simulink model "Citation_2017a"  (R2017a)
settings: Solver=ode5  StartTime=0.0  StopTime=inf  FixedStep=0.01  RelTol=1e-3  EnableMultiTasking=on
InitFcn:
  | initcit
values from neighbouring files (symbols this model uses):
  aeroinit = [dp_ini;inicoef('CX0');inicoef('CXa');inicoef('CXa2');inicoef('CXq')     ;inicoef('CXde');inicoef('CY0');inicoef('CYB');inicoef('CYp');inicoef('CYr')     ;inicoef('CYda');inicoef('CYdr');inicoef('CZ0');inicoef('CZa');inicoef('CZq')     ;inicoef('CZde');inicoef('Cl0');inicoef('ClB');inicoef('Clp');inicoef('Clr')     ;inicoef('Clda');inicoef('Cldr');inicoef('Cm0');inicoef('Cma');inicoef('Cmq')     ; ...(+113 chars)    [initcit.m]
  Clda_thresh = 3.410e-2/2    (= 0.01705)    [initcit.m]
  h_l_old = zeros(6,sample_size)    [initcit.m]
  h_m_old = zeros(4,sample_size)    [initcit.m]
  h_n_old = zeros(6,sample_size)    [initcit.m]
  h_X_old = zeros(5,sample_size)    [initcit.m]
  h_Y_old = zeros(6,sample_size)    [initcit.m]
  h_Z_old = zeros(4,sample_size)    [initcit.m]
  I = [massinit(5),0, -massinit(8);0, massinit(6),0;-massinit(8),0, massinit(7)]    [initcit.m]
  p_l = [inicoef('Cl0');inicoef('ClB');inicoef('Clp');inicoef('Clr')     ;inicoef('Clda');inicoef('Cldr')].*ones(6,sample_size)    [initcit.m]
  p_m = [inicoef('Cm0');inicoef('Cma');inicoef('Cmq')     ;inicoef('Cmde')].*ones(4,sample_size)    [initcit.m]
  p_n = [inicoef('Cn0');inicoef('CnB');inicoef('Cnp');inicoef('Cnr')     ;inicoef('Cnda');inicoef('Cndr')].*ones(6,sample_size)    [initcit.m]
  p_X = [inicoef('CX0');inicoef('CXa');inicoef('CXa2');inicoef('CXq')     ;inicoef('CXde')].*ones(5,sample_size)    [initcit.m]
  p_Y = [inicoef('CY0');inicoef('CYB');inicoef('CYp');inicoef('CYr')     ;inicoef('CYda');inicoef('CYdr')].*ones(6,sample_size)    [initcit.m]
  p_Z = [inicoef('CZ0');inicoef('CZa');inicoef('CZq')     ;inicoef('CZde')].*ones(4,sample_size)    [initcit.m]
  Pcov_l = 10000*eye(6)    [initcit.m]
  Pcov_m = 10000*eye(4)    [initcit.m]
  Pcov_n = 10000*eye(6)    [initcit.m]
  Pcov_X = 10000*eye(5)    [initcit.m]
  Pcov_Y = 10000*eye(6)    [initcit.m]
  Pcov_Z = 10000*eye(4)    [initcit.m]
  replay = 0    [initcit.m]
  T0 = 288.15    [rho_test.m]
  timeend = inputsim.data{1}.Values.Time(end)    [initcit.m]
  Vw915 = 0    [initcit.m]
  winddir = 45*(pi/180)    (= 0.785398163397)    [initcit.m]
  x0 = []    [cessnac550_3d_sfnc.m]    (also in sfunxyauto.m)
  y_l = zeros(1,sample_size)    [initcit.m]
  y_l_est_old = zeros(size(y_l))    [initcit.m]
  y_m = zeros(1,sample_size)    [initcit.m]
  y_m_est_old = zeros(size(y_m))    [initcit.m]
  y_n = zeros(1,sample_size)    [initcit.m]
  y_n_est_old = zeros(size(y_n))    [initcit.m]
  y_X = zeros(1,sample_size)    [initcit.m]
  y_X_est_old = zeros(size(y_X))    [initcit.m]
  y_Y = zeros(1,sample_size)    [initcit.m]
  y_Y_est_old = zeros(size(y_Y))    [initcit.m]
  y_Z = zeros(1,sample_size)    [initcit.m]
  y_Z_est_old = zeros(size(y_Z))    [initcit.m]
undefined symbols (not defined in the file or in its folder): chord, cv1, cv2, cv3, cv4, deltagmax1, deltagmax2, deltagmax3, deltagmax4, Deng, ealphag, ealphas, g0, hDME, hGS, kt1, kt2, kt3, lh, massinit, matbuaf, matdaf, matdam, matdbbf, matdeaf, matdgaf, matdqaf, matduaf, matdwaw, matedhr, mateif, matelhr, matemhr, matemv1, matemv2, matemve, matetam, mateuaf, matfaaf, matfaxl, matff, matibaf, matibmh, matipaf, matipmh, matiraf, matiuaf, matiwaf, matlaf, matlam, matleaf, matleam, matlgaf, matlqaf, matluaf, matmaaf, matmaam, matmaf, matmam, matmbbf ... (+74)
undefined symbols (not defined in the file): matibb
libraries: simulink x13, templibrary x6, vrlib x1
(part 3 of 7)

== system Citation_2017a/Cessna Citation 500/Citation model DASMAT/AIRCRAFT MODEL ==
  ua : Inport
  ut : Inport  Port=2
  massinit : Inport  Port=3
  Environment : Inport  Port=4
  AFM : Subsystem
  AIRDATA : Subsystem
  Demux : Demux  Outputs=[8 1]
  EFM : Subsystem
  EQM : Subsystem
  FM SORT : Subsystem
  GRAVITY : Subsystem
  LANDING GEAR : Subsystem
  OBSERVATIONS : Subsystem
  WIND/TURBULENCE : Subsystem
  x : Outport
  xdot : Outport  Port=2
  yatm : Outport  Port=3
  yad1 : Outport  Port=4
  yad2 : Outport  Port=5
  wind : Outport  Port=6
  gust : Outport  Port=7
  yacc : Outport  Port=8
  yfp : Outport  Port=9
  ys : Outport  Port=10
  FMa : Outport  Port=11
  FMag : Outport  Port=12
  FMt : Outport  Port=13
  ypp : Outport  Port=14
  wires:
  AFM/1(FMa) -> FM SORT/1(FMa), EQM/2(FMa)
  OBSERVATIONS/3(ys) -> ys/1
  OBSERVATIONS/2(yfp) -> yfp/1
  EQM/4(FMtot corrected) -> OBSERVATIONS/4(FMtot)
  EQM/3(yuvw) -> OBSERVATIONS/3(yuvw)
  EFM/1(FMt) -> FM SORT/3(FMt), FMt/1
  AFM/4(FMag) -> FM SORT/2(FMag), FMag/1
  ua/1 -> AFM/2(ua), LANDING GEAR/4(ua)
  ut/1 -> EFM/2(ut)
  OBSERVATIONS/1(yacc) -> yacc/1
  FM SORT/1(FMtot) -> EQM/1("FMtot ")
  EQM/5(FMa corrected) -> OBSERVATIONS/5(FMa), FMa/1
  AFM/2(FMadot) -> EQM/3(FMadot)
  AFM/3(FMbdot) -> EQM/4(FMbdot)
  GRAVITY/1(Fgr) -> FM SORT/4("Fgr "), OBSERVATIONS/6(Fgr)
  massinit/1 -> EFM/3(massinit), AFM/3(massinit), GRAVITY/2(massinit), EQM/5(massinit), OBSERVATIONS/7(massinit), LANDING GEAR/3(massinit)
  AIRDATA/3(yad2) -> EFM/6(yad2), AFM/5(yad2), yad2/1
  AIRDATA/2(yad1) -> AFM/4(yad1), EFM/5(yad1), yad1/1
  AIRDATA/1(yatm) -> yatm/1, GRAVITY/3(yatm), OBSERVATIONS/8(yatm), EFM/4(yatm), AFM/7(yatm)
  EQM/1(x) -> GRAVITY/1("x "), LANDING GEAR/1(x), EFM/1(x), AFM/1(x), WIND/TURBULENCE/1("x "), AIRDATA/1(x), x/1, OBSERVATIONS/1(x)
  WIND/TURBULENCE/1(wind) -> EQM/6(wind), wind/1
  EQM/2(xdot) -> xdot/1, OBSERVATIONS/2(xdot), LANDING GEAR/2(xdot)
  Environment/1 -> Demux/1
  Demux/1 -> gust/1, AFM/6(gust)
  Demux/2 -> AIRDATA/2(terrain elevation), LANDING GEAR/5(terr elev)  "terrain elevation"
  LANDING GEAR/1(Fmt) -> FM SORT/5(Fgear)
  EFM/2(ypp) -> ypp/1

== system Citation_2017a/Controllers/ANDI rotational rate controller/Linear Controller ==
  e_omega : Inport
  int reset : Inport  Port=2
  Demux : Demux  Outputs=3
  Mux : Mux  Inputs=3
  PID Controller : simulink/Continuous/PID Controller  Controller=PID  TimeDomain=Continuous-time  SampleTime=-1  IntegratorMethod=Forward Euler  FilterMethod=Forward Euler  Form=Parallel  UseFilter=on  ControllerParametersSource=internal  P=10  I=1  D=0  N=100  InitialConditionSource=internal  InitialConditionForIntegrator=0  InitialConditionForFilter=0  ExternalReset=rising  LimitOutput=off  UpperSaturationLimit=inf  LowerSaturationLimit=-inf  LinearizeAsGain=on  AntiWindupMode=none  Kb=1  TrackingMode=off  Kt=1  PParamMin=[]  PParamMax=[]  IParamMin=[]  IParamMax=[]  DParamMin=[]  DParamMax=[]  NParamMin=[]  NParamMax=[]  KbParamMin=[]  KbParamMax=[]  KtParamMin=[]  KtParamMax=[]  POutMin=[]  POutMax=[]  IOutMin=[]  IOutMax=[]  DOutMin=[]  DOutMax=[]  NOutMin=[]  NOutMax=[]  KbOutMin=[]  KbOutMax=[]  KtOutMin=[]  KtOutMax=[]  IntegratorOutMin=[]  IntegratorOutMax=[]  FilterOutMin=[]  FilterOutMax=[]  SumOutMin=[]  SumOutMax=[]  SumI1OutMin=[]  SumI1OutMax=[]  SumI2OutMin=[]  SumI2OutMax=[]  SumI3OutMin=[]  SumI3OutMax=[]  SumDOutMin=[]  SumDOutMax=[]  SaturationOutMin=[]  SaturationOutMax=[]  IntegratorContinuousStateAttributes=''  IntegratorStateMustResolveToSignalObject=off  IntegratorRTWStateStorageClass=Auto  FilterContinuousStateAttributes=''  FilterStateMustResolveToSignalObject=off  FilterRTWStateStorageClass=Auto  DifferentiatorICPrevScaledInput=0  DifferentiatorOutMin=[]  DifferentiatorOutMax=[]
  PID Controller1 : simulink/Continuous/PID Controller  Controller=PID  TimeDomain=Continuous-time  SampleTime=-1  IntegratorMethod=Forward Euler  FilterMethod=Forward Euler  Form=Parallel  UseFilter=on  ControllerParametersSource=internal  P=10  I=2  D=0  N=1  InitialConditionSource=internal  InitialConditionForIntegrator=0  InitialConditionForFilter=0  ExternalReset=rising  LimitOutput=off  UpperSaturationLimit=inf  LowerSaturationLimit=-inf  LinearizeAsGain=on  AntiWindupMode=none  Kb=1  TrackingMode=off  Kt=1  PParamMin=[]  PParamMax=[]  IParamMin=[]  IParamMax=[]  DParamMin=[]  DParamMax=[]  NParamMin=[]  NParamMax=[]  KbParamMin=[]  KbParamMax=[]  KtParamMin=[]  KtParamMax=[]  POutMin=[]  POutMax=[]  IOutMin=[]  IOutMax=[]  DOutMin=[]  DOutMax=[]  NOutMin=[]  NOutMax=[]  KbOutMin=[]  KbOutMax=[]  KtOutMin=[]  KtOutMax=[]  IntegratorOutMin=[]  IntegratorOutMax=[]  FilterOutMin=[]  FilterOutMax=[]  SumOutMin=[]  SumOutMax=[]  SumI1OutMin=[]  SumI1OutMax=[]  SumI2OutMin=[]  SumI2OutMax=[]  SumI3OutMin=[]  SumI3OutMax=[]  SumDOutMin=[]  SumDOutMax=[]  SaturationOutMin=[]  SaturationOutMax=[]  IntegratorContinuousStateAttributes=''  IntegratorStateMustResolveToSignalObject=off  IntegratorRTWStateStorageClass=Auto  FilterContinuousStateAttributes=''  FilterStateMustResolveToSignalObject=off  FilterRTWStateStorageClass=Auto  DifferentiatorICPrevScaledInput=0  DifferentiatorOutMin=[]  DifferentiatorOutMax=[]
  PID Controller2 : simulink/Continuous/PID Controller  Controller=PID  TimeDomain=Continuous-time  SampleTime=-1  IntegratorMethod=Forward Euler  FilterMethod=Forward Euler  Form=Parallel  UseFilter=on  ControllerParametersSource=internal  P=8  I=2  D=0  N=1  InitialConditionSource=internal  InitialConditionForIntegrator=0  InitialConditionForFilter=0  ExternalReset=rising  LimitOutput=off  UpperSaturationLimit=inf  LowerSaturationLimit=-inf  LinearizeAsGain=on  AntiWindupMode=none  Kb=1  TrackingMode=off  Kt=1  PParamMin=[]  PParamMax=[]  IParamMin=[]  IParamMax=[]  DParamMin=[]  DParamMax=[]  NParamMin=[]  NParamMax=[]  KbParamMin=[]  KbParamMax=[]  KtParamMin=[]  KtParamMax=[]  POutMin=[]  POutMax=[]  IOutMin=[]  IOutMax=[]  DOutMin=[]  DOutMax=[]  NOutMin=[]  NOutMax=[]  KbOutMin=[]  KbOutMax=[]  KtOutMin=[]  KtOutMax=[]  IntegratorOutMin=[]  IntegratorOutMax=[]  FilterOutMin=[]  FilterOutMax=[]  SumOutMin=[]  SumOutMax=[]  SumI1OutMin=[]  SumI1OutMax=[]  SumI2OutMin=[]  SumI2OutMax=[]  SumI3OutMin=[]  SumI3OutMax=[]  SumDOutMin=[]  SumDOutMax=[]  SaturationOutMin=[]  SaturationOutMax=[]  IntegratorContinuousStateAttributes=''  IntegratorStateMustResolveToSignalObject=off  IntegratorRTWStateStorageClass=Auto  FilterContinuousStateAttributes=''  FilterStateMustResolveToSignalObject=off  FilterRTWStateStorageClass=Auto  DifferentiatorICPrevScaledInput=0  DifferentiatorOutMin=[]  DifferentiatorOutMax=[]
  v : Outport
  wires:
  Demux/1 -> PID Controller1/1
  PID Controller2/1 -> Mux/3  "vr"
  PID Controller/1 -> Mux/2  "vq"
  Demux/3 -> PID Controller2/1
  PID Controller1/1 -> Mux/1  "vp"
  Demux/2 -> PID Controller/1
  Mux/1 -> v/1
  e_omega/1 -> Demux/1
  int reset/1 -> PID Controller/2, PID Controller2/2, PID Controller1/2

== system Citation_2017a/Controllers/Default Actuator Control/Yaw damper1 ==
  state : Inport
  inputs : Inport  Port=2
  Gain : Gain  SaturateOnIntegerOverflow=on  OutDataTypeStr=Inherit: Same as input  ParamDataTypeStr=Inherit: Same as input
  Washout : TransferFcn  Numerator=[1 0]  Denominator=[1 1/4]
  dr : Gain  Gain=[0 0 1 0 0 0 0 0 0 0]  SaturateOnIntegerOverflow=on  OutDataTypeStr=Inherit: Same as input  ParamDataTypeStr=Inherit: Same as input
  not used : Terminator
  r  sel : Selector  IndexOptions=Index vector (dialog)  Indices=[3]  OutputSizes=1
  controller output : Outport
  wires:
  Washout/1 -> Gain/1
  dr/1 -> controller output/1
  state/1 -> r  sel/1
  r  sel/1 -> Washout/1  "r"
  inputs/1 -> not used/1
  Gain/1 -> dr/1

== system Citation_2017a/Controllers/Default Actuator Control/auto throttle1 ==
  state : Inport
  inputs : Inport  Port=2
  Gain : Gain  Gain=0.5  SaturateOnIntegerOverflow=on  OutDataTypeStr=Inherit: Same as input  ParamDataTypeStr=Inherit: Same as input
  Saturation : Saturate  UpperLimit=1.0  LowerLimit=0.0
  Sum : Sum  Inputs=+-|  SaturateOnIntegerOverflow=on
  VTAS ref (trim value) : Constant  Value=x0(4)
  VTAS sel : Selector  IndexOptions=Index vector (dialog)  Indices=[4]  OutputSizes=1
  controller output is later added to pilot input! : Sum  Inputs=|+-  SaturateOnIntegerOverflow=on
  pla1&2 : Gain  Gain=[0 0 0 0 0 0 0 0 1 1]  SaturateOnIntegerOverflow=on  OutDataTypeStr=Inherit: Same as input  ParamDataTypeStr=Inherit: Same as input
  pla1&2 as well : Gain  Gain=[0 0 0 0 0 0 0 0 1 1]  SaturateOnIntegerOverflow=on  OutDataTypeStr=Inherit: Same as input  ParamDataTypeStr=Inherit: Same as input
  controller output : Outport
  wires:
  inputs/1 -> pla1&2 as well/1
  state/1 -> VTAS sel/1
  VTAS sel/1 -> Sum/2  "VTAS"
  VTAS ref (trim value)/1 -> Sum/1
  Sum/1 -> Gain/1
  pla1&2/1 -> controller output is later added to pilot input!/1
  Gain/1 -> Saturation/1
  controller output is later added to pilot input!/1 -> controller output/1
  Saturation/1 -> pla1&2/1
  pla1&2 as well/1 -> controller output is later added to pilot input!/2

== system Citation_2017a/Controllers/INDI rotational rate controller/Linear Controller ==
  e_omega : Inport
  int reset : Inport  Port=2
  Demux : Demux  Outputs=3
  Mux : Mux  Inputs=3
  PID Controller : simulink/Continuous/PID Controller  Controller=PID  TimeDomain=Continuous-time  SampleTime=-1  IntegratorMethod=Forward Euler  FilterMethod=Forward Euler  Form=Parallel  UseFilter=on  ControllerParametersSource=internal  P=10  I=1  D=0  N=100  InitialConditionSource=internal  InitialConditionForIntegrator=0  InitialConditionForFilter=0  ExternalReset=rising  LimitOutput=off  UpperSaturationLimit=inf  LowerSaturationLimit=-inf  LinearizeAsGain=on  AntiWindupMode=none  Kb=1  TrackingMode=off  Kt=1  PParamMin=[]  PParamMax=[]  IParamMin=[]  IParamMax=[]  DParamMin=[]  DParamMax=[]  NParamMin=[]  NParamMax=[]  KbParamMin=[]  KbParamMax=[]  KtParamMin=[]  KtParamMax=[]  POutMin=[]  POutMax=[]  IOutMin=[]  IOutMax=[]  DOutMin=[]  DOutMax=[]  NOutMin=[]  NOutMax=[]  KbOutMin=[]  KbOutMax=[]  KtOutMin=[]  KtOutMax=[]  IntegratorOutMin=[]  IntegratorOutMax=[]  FilterOutMin=[]  FilterOutMax=[]  SumOutMin=[]  SumOutMax=[]  SumI1OutMin=[]  SumI1OutMax=[]  SumI2OutMin=[]  SumI2OutMax=[]  SumI3OutMin=[]  SumI3OutMax=[]  SumDOutMin=[]  SumDOutMax=[]  SaturationOutMin=[]  SaturationOutMax=[]  IntegratorContinuousStateAttributes=''  IntegratorStateMustResolveToSignalObject=off  IntegratorRTWStateStorageClass=Auto  FilterContinuousStateAttributes=''  FilterStateMustResolveToSignalObject=off  FilterRTWStateStorageClass=Auto  DifferentiatorICPrevScaledInput=0  DifferentiatorOutMin=[]  DifferentiatorOutMax=[]
  PID Controller1 : simulink/Continuous/PID Controller  Controller=PID  TimeDomain=Continuous-time  SampleTime=-1  IntegratorMethod=Forward Euler  FilterMethod=Forward Euler  Form=Parallel  UseFilter=on  ControllerParametersSource=internal  P=10  I=2  D=0  N=1  InitialConditionSource=internal  InitialConditionForIntegrator=0  InitialConditionForFilter=0  ExternalReset=rising  LimitOutput=off  UpperSaturationLimit=inf  LowerSaturationLimit=-inf  LinearizeAsGain=on  AntiWindupMode=none  Kb=1  TrackingMode=off  Kt=1  PParamMin=[]  PParamMax=[]  IParamMin=[]  IParamMax=[]  DParamMin=[]  DParamMax=[]  NParamMin=[]  NParamMax=[]  KbParamMin=[]  KbParamMax=[]  KtParamMin=[]  KtParamMax=[]  POutMin=[]  POutMax=[]  IOutMin=[]  IOutMax=[]  DOutMin=[]  DOutMax=[]  NOutMin=[]  NOutMax=[]  KbOutMin=[]  KbOutMax=[]  KtOutMin=[]  KtOutMax=[]  IntegratorOutMin=[]  IntegratorOutMax=[]  FilterOutMin=[]  FilterOutMax=[]  SumOutMin=[]  SumOutMax=[]  SumI1OutMin=[]  SumI1OutMax=[]  SumI2OutMin=[]  SumI2OutMax=[]  SumI3OutMin=[]  SumI3OutMax=[]  SumDOutMin=[]  SumDOutMax=[]  SaturationOutMin=[]  SaturationOutMax=[]  IntegratorContinuousStateAttributes=''  IntegratorStateMustResolveToSignalObject=off  IntegratorRTWStateStorageClass=Auto  FilterContinuousStateAttributes=''  FilterStateMustResolveToSignalObject=off  FilterRTWStateStorageClass=Auto  DifferentiatorICPrevScaledInput=0  DifferentiatorOutMin=[]  DifferentiatorOutMax=[]
  PID Controller2 : simulink/Continuous/PID Controller  Controller=PID  TimeDomain=Continuous-time  SampleTime=-1  IntegratorMethod=Forward Euler  FilterMethod=Forward Euler  Form=Parallel  UseFilter=on  ControllerParametersSource=internal  P=8  I=2  D=0  N=1  InitialConditionSource=internal  InitialConditionForIntegrator=0  InitialConditionForFilter=0  ExternalReset=rising  LimitOutput=off  UpperSaturationLimit=inf  LowerSaturationLimit=-inf  LinearizeAsGain=on  AntiWindupMode=none  Kb=1  TrackingMode=off  Kt=1  PParamMin=[]  PParamMax=[]  IParamMin=[]  IParamMax=[]  DParamMin=[]  DParamMax=[]  NParamMin=[]  NParamMax=[]  KbParamMin=[]  KbParamMax=[]  KtParamMin=[]  KtParamMax=[]  POutMin=[]  POutMax=[]  IOutMin=[]  IOutMax=[]  DOutMin=[]  DOutMax=[]  NOutMin=[]  NOutMax=[]  KbOutMin=[]  KbOutMax=[]  KtOutMin=[]  KtOutMax=[]  IntegratorOutMin=[]  IntegratorOutMax=[]  FilterOutMin=[]  FilterOutMax=[]  SumOutMin=[]  SumOutMax=[]  SumI1OutMin=[]  SumI1OutMax=[]  SumI2OutMin=[]  SumI2OutMax=[]  SumI3OutMin=[]  SumI3OutMax=[]  SumDOutMin=[]  SumDOutMax=[]  SaturationOutMin=[]  SaturationOutMax=[]  IntegratorContinuousStateAttributes=''  IntegratorStateMustResolveToSignalObject=off  IntegratorRTWStateStorageClass=Auto  FilterContinuousStateAttributes=''  FilterStateMustResolveToSignalObject=off  FilterRTWStateStorageClass=Auto  DifferentiatorICPrevScaledInput=0  DifferentiatorOutMin=[]  DifferentiatorOutMax=[]
  v : Outport
  wires:
  Demux/1 -> PID Controller1/1
  PID Controller2/1 -> Mux/3  "vr"
  PID Controller/1 -> Mux/2  "vq"
  Demux/3 -> PID Controller2/1
  PID Controller1/1 -> Mux/1  "vp"
  Demux/2 -> PID Controller/1
  Mux/1 -> v/1
  e_omega/1 -> Demux/1
  int reset/1 -> PID Controller/2, PID Controller2/2, PID Controller1/2

== system Citation_2017a/Flight Monitoring/3D Display/Position ==
  Mux2 : Mux  Inputs=3
  x : Constant  Value=0
  y : Constant  Value=0
  z : Constant  Value=0
  Out1 : Outport
  wires:
  y/1 -> Mux2/2
  z/1 -> Mux2/3
  x/1 -> Mux2/1
  Mux2/1 -> Out1/1

== system Citation_2017a/Pilot/Joystick/DualShock ==
  note: Apply Dead zone
  note: Currently configured for a Sony Dualshock 3 Playstation 3 Controller
  JoyStick input : Inport
  "Add deadzone " : Subsystem
  Add deadzone 1 : Subsystem
  Add deadzone 2 : Subsystem
  Add deadzone 3 : Subsystem
  Constant{,1..3} (4 alike) : Constant  Value=0
  Constant{4..7} (4 alike) : Constant  Value=0.05
  Dead Zone{,1..3} (4 alike) : DeadZone  LowerValue=-0.05  UpperValue=0.05  SaturateOnIntegerOverflow=on
  Demux : Demux  Outputs=[5 10]
  Demux1 : Demux  Outputs=5
  Demux2 : Demux  Outputs=[2 1 7]
  Display{,1..3} (4 alike) : Display
  Gain{,1..3} (4 alike) : Gain  Gain=-1  SaturateOnIntegerOverflow=on  OutDataTypeStr=Inherit: Same as input  ParamDataTypeStr=Inherit: Same as input
  Gain11 : Gain  Gain=pi/180  SaturateOnIntegerOverflow=on  OutDataTypeStr=Inherit: Same as input  ParamDataTypeStr=Inherit: Same as input
  Gain4 : Gain  Gain=37.24  SaturateOnIntegerOverflow=on  OutDataTypeStr=Inherit: Same as input  ParamDataTypeStr=Inherit: Same as input
  Gain5 : Gain  Gain=20  SaturateOnIntegerOverflow=on  OutDataTypeStr=Inherit: Same as input  ParamDataTypeStr=Inherit: Same as input
  Gain6 : Gain  SaturateOnIntegerOverflow=on  OutDataTypeStr=Inherit: Same as input  ParamDataTypeStr=Inherit: Same as input
  Gain7 : Gain  Gain=22  SaturateOnIntegerOverflow=on  OutDataTypeStr=Inherit: Same as input  ParamDataTypeStr=Inherit: Same as input
  Gain8 : Gain  Gain=pi/180  SaturateOnIntegerOverflow=on  OutDataTypeStr=Inherit: Same as input  ParamDataTypeStr=Inherit: Same as input
  Gain9 : Gain  Gain=pi/180  SaturateOnIntegerOverflow=on  OutDataTypeStr=Inherit: Same as input  ParamDataTypeStr=Inherit: Same as input
  Mux : Mux  Inputs=5
  Sum{,1..3} (4 alike) : Sum  Inputs=-+|  SaturateOnIntegerOverflow=on
  Terminator : Terminator
  Terminator1 : Terminator
  Terminator2 : Terminator
  "Model Input " : Outport
  wires:
  Gain3/1 -> Gain7/1
  Constant4/1 -> "Add deadzone "/1("Value ")
  Gain4/1 -> Gain8/1
  Constant5/1 -> Add deadzone 3/1("Value ")
  Constant/1 -> Sum/1
  Sum3/1 -> Dead Zone2/1
  "Add deadzone "/1(Out1) -> Gain/1
  Demux1/3 -> Terminator/1
  Demux1/4 -> Sum3/2
  Dead Zone/1 -> "Add deadzone "/2("Input ")
  Sum2/1 -> Dead Zone3/1
  Gain8/1 -> Mux/1, Display/1
  Dead Zone1/1 -> Add deadzone 1/2("Input ")
  Demux1/5 -> Sum1/2
  Add deadzone 1/1(Out1) -> Gain1/1
  Add deadzone 3/1(Out1) -> Gain3/1
  Constant1/1 -> Sum1/1
  Demux1/2 -> Sum2/2
  Gain5/1 -> Gain9/1
  Gain11/1 -> Mux/4, Display3/1
  Constant3/1 -> Sum3/1
  Gain1/1 -> Gain5/1
  Dead Zone2/1 -> Add deadzone 3/2("Input ")
  Add deadzone 2/1(Out1) -> Gain2/1
  Gain/1 -> Gain4/1
  Dead Zone3/1 -> Add deadzone 2/2("Input ")
  Sum/1 -> Dead Zone/1
  Gain9/1 -> Mux/2, Display2/1
  Constant7/1 -> Add deadzone 1/1("Value ")
  Constant6/1 -> Add deadzone 2/1("Value ")
  Sum1/1 -> Dead Zone1/1
  Gain6/1 -> Mux/3, Display1/1
  Gain7/1 -> Gain11/1
  Demux1/1 -> Sum/2
  Constant2/1 -> Sum2/1
  Gain2/1 -> Gain6/1
  JoyStick input/1 -> Demux/1
  Demux2/3 -> Terminator2/1
  Demux/2 -> Demux2/1  "buttons"
  Demux2/1 -> Terminator1/1
  Demux/1 -> Demux1/1
  Mux/1 -> "Model Input "/1
  Demux2/2 -> Mux/5

== system Citation_2017a/Pilot/Joystick/Logitech 3D Pro ==
  note: Apply real actuator limits
  note: Normalize inputs
  note: Apply Dead zone
  note: apply real limits
      | [deg]
      | [%]
  note: normalize inputs
      | aileron [-1,0,1] left+
      | elevator [-1,0,1] forward+
      | rudder [-1,0,1] left+
      | throttle [-1,0,1] forward+
  note: Convert to radians
      | [rad]
      | [%]
  note: raw inputs
      | aileron [-0.6328,0.014,0.72] right+
      | elevator [-0.6973,-0.033,0.5725] backwards+
      | throttle [-0.6407,0,0.5317]bacwards+
      | rudder [-0.56,0.127,0.73] right+
  note: Currently configured for a Logitech Xtreme 3D Pro Joystick
  "JoyStick Input " : Inport
  Constant{,1..3} (4 alike) : Constant  Value=0
  Dead Zone : DeadZone  LowerValue=-0.2  UpperValue=0.2  SaturateOnIntegerOverflow=on
  Dead Zone1 : DeadZone  LowerValue=-0.008  UpperValue=0.008  SaturateOnIntegerOverflow=on
  Dead Zone2 : DeadZone  LowerValue=-0.05  UpperValue=0.05  SaturateOnIntegerOverflow=on
  Dead Zone3 : DeadZone  LowerValue=0  UpperValue=0  SaturateOnIntegerOverflow=on
  Demux : Demux  Outputs=[1 1 2 1 1 2 1 1 1 1]
  Demux1 : Demux
  Demux2 : Demux  Outputs=[4 12]
  Gain : Gain  Gain=-1/0.8  SaturateOnIntegerOverflow=on  OutDataTypeStr=Inherit: Same as input  ParamDataTypeStr=Inherit: Same as input
  Gain1 : Gain  Gain=-1/0.992  SaturateOnIntegerOverflow=on  OutDataTypeStr=Inherit: Same as input  ParamDataTypeStr=Inherit: Same as input
  Gain11 : Gain  Gain=pi/180  SaturateOnIntegerOverflow=on  OutDataTypeStr=Inherit: Same as input  ParamDataTypeStr=Inherit: Same as input
  Gain2 : Gain  Gain=-1  SaturateOnIntegerOverflow=on  OutDataTypeStr=Inherit: Same as input  ParamDataTypeStr=Inherit: Same as input
  Gain3 : Gain  Gain=-1/0.95  SaturateOnIntegerOverflow=on  OutDataTypeStr=Inherit: Same as input  ParamDataTypeStr=Inherit: Same as input
  Gain4 : Gain  Gain=37.24  SaturateOnIntegerOverflow=on  OutDataTypeStr=Inherit: Same as input  ParamDataTypeStr=Inherit: Same as input
  Gain5 : Gain  Gain=20  SaturateOnIntegerOverflow=on  OutDataTypeStr=Inherit: Same as input  ParamDataTypeStr=Inherit: Same as input
  Gain6 : Gain  SaturateOnIntegerOverflow=on  OutDataTypeStr=Inherit: Same as input  ParamDataTypeStr=Inherit: Same as input
  Gain7 : Gain  Gain=22  SaturateOnIntegerOverflow=on  OutDataTypeStr=Inherit: Same as input  ParamDataTypeStr=Inherit: Same as input
  Gain8 : Gain  Gain=pi/180  SaturateOnIntegerOverflow=on  OutDataTypeStr=Inherit: Same as input  ParamDataTypeStr=Inherit: Same as input
  Gain9 : Gain  Gain=pi/180  SaturateOnIntegerOverflow=on  OutDataTypeStr=Inherit: Same as input  ParamDataTypeStr=Inherit: Same as input
  Mux : Mux  Inputs=11
  Sum{,1..3} (4 alike) : Sum  Inputs=-+|  SaturateOnIntegerOverflow=on
  Terminator1 : Terminator
  Terminator2 : Terminator
  Terminator3 : Terminator
  Model Input : Outport
  wires:
  Constant1/1 -> Sum1/1
  Sum2/1 -> Dead Zone3/1
  Sum/1 -> Dead Zone/1
  Dead Zone/1 -> Gain/1
  Dead Zone2/1 -> Gain3/1
  Dead Zone3/1 -> Gain2/1
  Gain5/1 -> Gain9/1
  Gain7/1 -> Gain11/1
  Dead Zone1/1 -> Gain1/1
  Constant2/1 -> Sum2/1
  Sum1/1 -> Dead Zone1/1
  Sum3/1 -> Dead Zone2/1
  Gain4/1 -> Gain8/1
  Demux1/1 -> Sum/2
  Gain1/1 -> Gain5/1
  Constant/1 -> Sum/1
  Demux2/1 -> Demux1/1  "axes"
  Gain3/1 -> Gain7/1
  Constant3/1 -> Sum3/1
  Gain2/1 -> Gain6/1
  Gain/1 -> Gain4/1
  Demux1/3 -> Sum3/2
  Demux1/2 -> Sum1/2
  Demux1/4 -> Sum2/2
  Gain9/1 -> Mux/2  "elevator"
  Gain6/1 -> Mux/3  "thrust"
  Demux/6 -> Terminator2/1
  Demux/1 -> Terminator1/1
  Demux/4 -> Mux/5  "failure button"
  Demux2/2 -> Demux/1  "buttons"
  "JoyStick Input "/1 -> Demux2/1
  Mux/1 -> Model Input/1
  Gain8/1 -> Mux/1  "aileron"
  Gain11/1 -> Mux/4  "rudder"
  Demux/9 -> Mux/8  "Default mode"
  Demux/7 -> Mux/6  "classical rate toggle"
  Demux/10 -> Mux/9  "NDI toggle"
  Demux/8 -> Mux/7  "INDI toggle"
  Demux/3 -> Terminator3/1
  Demux/2 -> Mux/10  "Manual integral reset"
  Demux/5 -> Mux/11  "AT toggle"

== system Citation_2017a/Pilot/Joystick/Stop sim when replay has ended ==
  In1 : Inport
  Clock : Clock
      settings: Decimation=2
  Constant2 : Constant  Value=inf
  Constant3 : Constant  Value=timeend
  Display : Display
  Fcn : Fcn  Expr=u<0
  Stop Simulation : Stop
  Sum1 : Sum  Inputs=|+-
  Switch : Switch  Criteria=u2 > Threshold
  wires:
  Switch/1 -> Sum1/1
  Constant3/1 -> Switch/1
  Fcn/1 -> Stop Simulation/1
  Sum1/1 -> Display/1, Fcn/1
  In1/1 -> Switch/2
  Constant2/1 -> Switch/3
  Clock/1 -> Sum1/2

== system Citation_2017a/Pilot/Joystick/load pre-recorded inputs ==
  From Workspace : FromWorkspace  Commented=on  VariableName=inputsim.data{1}.Values  SampleTime=0
  From Workspace1 : FromWorkspace  Commented=on  VariableName=inputsim.data{3}.Values  SampleTime=0
  From Workspace10 : FromWorkspace  Commented=on  VariableName=inputsim.data{12}.Values  SampleTime=0
  From Workspace11 : FromWorkspace  Commented=on  VariableName=inputsim.data{10}.Values  SampleTime=0
  From Workspace12 : FromWorkspace  Commented=on  VariableName=inputsim.data{11}.Values  SampleTime=0
  From Workspace13 : FromWorkspace  Commented=on  VariableName=inputsim.data{14}.Values  SampleTime=0
  From Workspace14 : FromWorkspace  Commented=on  VariableName=inputsim.data{13}.Values  SampleTime=0
  From Workspace15 : FromWorkspace  Commented=on  VariableName=inputsim.data{16}.Values  SampleTime=0
  From Workspace16 : FromWorkspace  VariableName=joydata  SampleTime=0
  From Workspace2 : FromWorkspace  Commented=on  VariableName=inputsim.data{4}.Values  SampleTime=0
  From Workspace3 : FromWorkspace  Commented=on  VariableName=inputsim.data{5}.Values  SampleTime=0
  From Workspace4 : FromWorkspace  Commented=on  VariableName=inputsim.data{6}.Values  SampleTime=0
  From Workspace5 : FromWorkspace  Commented=on  VariableName=inputsim.data{7}.Values  SampleTime=0
  From Workspace6 : FromWorkspace  Commented=on  VariableName=inputsim.data{8}.Values  SampleTime=0
  From Workspace7 : FromWorkspace  Commented=on  VariableName=inputsim.data{9}.Values  SampleTime=0
  From Workspace8 : FromWorkspace  Commented=on  VariableName=inputsim.data{2}.Values  SampleTime=0
  From Workspace9 : FromWorkspace  Commented=on  VariableName=inputsim.data{15}.Values  SampleTime=0
  Mux : Mux  Commented=on  Inputs=16
  Out1 : Outport
  wires:
  From Workspace/1 -> Mux/1
  From Workspace8/1 -> Mux/2
  From Workspace1/1 -> Mux/3
  From Workspace2/1 -> Mux/4
  From Workspace3/1 -> Mux/5
  From Workspace4/1 -> Mux/6
  From Workspace5/1 -> Mux/7
  From Workspace6/1 -> Mux/8
  From Workspace7/1 -> Mux/9
  From Workspace11/1 -> Mux/10
  From Workspace12/1 -> Mux/11
  From Workspace10/1 -> Mux/12
  From Workspace14/1 -> Mux/13
  From Workspace13/1 -> Mux/14
  From Workspace9/1 -> Mux/15
  From Workspace15/1 -> Mux/16
  From Workspace16/1 -> Out1/1

== system Citation_2017a/Pilot/Select new mode/Triggered Subsystem ==
  note: default mode is the initial condition
  triggers : Inport
  Trigger : TriggerPort  TriggerType=either  VariantControl=Variant
  MATLAB Function : MATLAB Function  TreatAsAtomicUnit=on
  Memory : Memory  X0=zeros(4,1)  InheritSampleTime=on
  Memory1 : Memory  X0=4  InheritSampleTime=on
  index : Outport
  wires:
  triggers/1 -> MATLAB Function/2(triggers)
  MATLAB Function/1(index) -> Memory1/1, index/1
  MATLAB Function/2(triggers_pref) -> Memory/1
  Memory/1 -> MATLAB Function/3("triggers_pref ")
  Memory1/1 -> MATLAB Function/1("index ")

== system Citation_2017a/Cessna Citation 500/Citation model DASMAT/AIRCRAFT MODEL/AFM ==
  x : Inport
  ua : Inport  Port=2
  massinit : Inport  Port=3
  yad1 : Inport  Port=4
  yad2 : Inport  Port=5
  gust : Inport  Port=6
  yatm : Inport  Port=7
  Aero axes-cg transformation : Subsystem
  Aeromod : Subsystem
  FMaerodims : Subsystem
  FMgustdims : Subsystem
  Gust axes-cg transformation : Subsystem
  FMa : Outport
  FMadot : Outport  Port=2
  FMbdot : Outport  Port=3
  FMag : Outport  Port=4
  wires:
  FMaerodims/3(FMbdot) -> FMbdot/1
  FMgustdims/1(FMag) -> FMag/1
  FMaerodims/2(FMadot) -> FMadot/1
  FMaerodims/1(FMa) -> FMa/1
  ua/1 -> Aeromod/2(ua)
  yad2/1 -> Aeromod/5(yad2)
  gust/1 -> Aeromod/6(gust)
  Aero axes-cg transformation/1(Ca) -> FMaerodims/1(Ca)
  Aero axes-cg transformation/2(Cadot) -> FMaerodims/2(Cadot)
  Aero axes-cg transformation/3(Cbdot) -> FMaerodims/3(Cbdot)
  Gust axes-cg transformation/1(Cag) -> FMgustdims/1(Cag)
  yad1/1 -> FMaerodims/5(yad1), FMgustdims/2(yad1), Aeromod/4(yad1)
  massinit/1 -> Aero axes-cg transformation/5(massinit), Gust axes-cg transformation/3(massinit), Aeromod/3(massinit)
  Aeromod/1(Ca) -> Aero axes-cg transformation/1(Ca model)
  Aeromod/2(Cadot) -> Aero axes-cg transformation/2(Cadot model)
  Aeromod/3(Cbdot) -> Aero axes-cg transformation/3(Cbdot model)
  Aeromod/4(Cag) -> Gust axes-cg transformation/1(Cag model)
  x/1 -> Aero axes-cg transformation/4("x "), Gust axes-cg transformation/2("x "), FMaerodims/4(x), Aeromod/1(x)
  yatm/1 -> Aeromod/7(yatm)

== system Citation_2017a/Cessna Citation 500/Citation model DASMAT/AIRCRAFT MODEL/AIRDATA ==
  x : Inport
  terrain elevation : Inport  Port=2
  Demux : Demux  Outputs=[8 2 8]
  Demux1 : Demux  Outputs=[5 1 2]
  Mux : Mux  Inputs=[5 1 2]
  Sum : Sum  Inputs=-+|  SaturateOnIntegerOverflow=on
  airdata : S-Function  FunctionName=ac_atmos  SFunctionDeploymentMode=off  EnableBusSupport=off
  yatm : Outport
  yad1 : Outport  Port=2
  yad2 : Outport  Port=3
  wires:
  x/1 -> airdata/1
  airdata/1 -> Demux/1
  Demux/2 -> yad1/1
  Demux/3 -> yad2/1
  Demux/1 -> Demux1/1
  Mux/1 -> yatm/1
  Demux1/1 -> Mux/1
  Demux1/3 -> Mux/3
  Demux1/2 -> Sum/2
  Sum/1 -> Mux/2
  terrain elevation/1 -> Sum/1

== system Citation_2017a/Cessna Citation 500/Citation model DASMAT/AIRCRAFT MODEL/EFM ==
  x : Inport
  ut : Inport  Port=2
  massinit : Inport  Port=3
  yatm : Inport  Port=4
  yad1 : Inport  Port=5
  yad2 : Inport  Port=6
  Engine axes-cg transformation : Subsystem
  Engmod : Subsystem
  FMt : Outport
  ypp : Outport  Port=2
  wires:
  massinit/1 -> Engine axes-cg transformation/3(massinit)
  Engine axes-cg transformation/1(FMt) -> FMt/1
  ut/1 -> Engmod/2(ut)
  yatm/1 -> Engmod/3(yatm)
  yad2/1 -> Engmod/5(yad2)
  x/1 -> Engine axes-cg transformation/2("x "), Engmod/1(x)
  yad1/1 -> Engmod/4(yad1)
  Engmod/1(FMt) -> Engine axes-cg transformation/1(FMt model)
  Engmod/2(ypp) -> ypp/1

== system Citation_2017a/Cessna Citation 500/Citation model DASMAT/AIRCRAFT MODEL/EQM ==
  "FMtot " : Inport
  FMa : Inport  Port=2
  FMadot : Inport  Port=3
  FMbdot : Inport  Port=4
  massinit : Inport  Port=5
  wind : Inport  Port=6
  Atan2 : Trigonometry  Commented=on  Operator=atan2
  CFMa correction : Subsystem
  Demux : Demux  Commented=on  Outputs=[9 1 1 1]
  Gain : Gain  Commented=on  Gain=180/pi
  Heading : Scope  Commented=on
  Integrator : Integrator  InitialCondition=x0
  State Derivatives : Subsystem
  Terminator : Terminator  Commented=on
  x : Outport
  xdot : Outport  Port=2
  yuvw : Outport  Port=3
  FMtot corrected : Outport  Port=4
  FMa corrected : Outport  Port=5
  wires:
  State Derivatives/2(yuvw) -> yuvw/1
  State Derivatives/3(FMtot corrected) -> FMtot corrected/1
  FMa/1 -> CFMa correction/2(FMa)
  State Derivatives/1(xdot) -> Demux/1, xdot/1, CFMa correction/1(xdot), Integrator/1
  CFMa correction/1(FMa corrected) -> FMa corrected/1
  massinit/1 -> State Derivatives/5(massinit)
  "FMtot "/1 -> State Derivatives/2(FMtot)
  FMadot/1 -> CFMa correction/3(FMadot), State Derivatives/3(FMadot)
  FMbdot/1 -> CFMa correction/4(FMbdot), State Derivatives/4(FMbdot)
  Integrator/1 -> State Derivatives/1(x), x/1
  wind/1 -> State Derivatives/6(wind)
  Demux/1 -> Terminator/1
  Demux/4 -> Atan2/1
  Atan2/1 -> Gain/1
  Gain/1 -> Heading/1
  Demux/3 -> Atan2/2

== system Citation_2017a/Cessna Citation 500/Citation model DASMAT/AIRCRAFT MODEL/FM SORT ==
  FMa : Inport
  FMag : Inport  Port=2
  FMt : Inport  Port=3
  "Fgr " : Inport  Port=4
  Fgear : Inport  Port=5
  Mux : Mux  Inputs=[12 12]
  Sum : Sum  Inputs=+++++  SaturateOnIntegerOverflow=on  InputSameDT=on  OutDataTypeStr=Inherit: Same as first input
  Sum1 : Sum  Inputs=++++  SaturateOnIntegerOverflow=on  InputSameDT=on  OutDataTypeStr=Inherit: Same as first input
  aero : Demux  Outputs=[12 12]
  engine : Demux  Outputs=[12 12]
  gear : Demux  Outputs=[12 12]
  gust : Demux  Outputs=[12 12]
  FMtot : Outport
  wires:
  FMt/1 -> engine/1
  FMa/1 -> aero/1
  FMag/1 -> gust/1
  gust/2 -> Sum1/2
  Sum1/1 -> Mux/2
  engine/2 -> Sum1/3
  aero/2 -> Sum1/1
  gust/1 -> Sum/2
  engine/1 -> Sum/3
  Sum/1 -> Mux/1
  "Fgr "/1 -> Sum/4
  aero/1 -> Sum/1
  Mux/1 -> FMtot/1
  Fgear/1 -> gear/1
  gear/1 -> Sum/5
  gear/2 -> Sum1/4

== system Citation_2017a/Cessna Citation 500/Citation model DASMAT/AIRCRAFT MODEL/GRAVITY ==
  "x " : Inport
  massinit : Inport  Port=2
  yatm : Inport  Port=3
  Fgr transformation : S-Function  FunctionName=ac_axes  Parameters=3  SFunctionDeploymentMode=off  EnableBusSupport=off
  Mux : Mux  Inputs=[12 3]
  Mux1 : Mux  Inputs=3
  Terminator_{1..9} (9 alike) : Terminator
  W : Product  SaturateOnIntegerOverflow=on  InputSameDT=on  OutDataTypeStr=Inherit: Same as first input
  atmosphere : Demux  Outputs=8
  mass cg inertia : Demux  Outputs=[1 3 4]
  zero : Constant  Value=0
  Fgr : Outport
  wires:
  mass cg inertia/3 -> Terminator_9/1
  mass cg inertia/2 -> Terminator_8/1
  atmosphere/8 -> Terminator_7/1
  atmosphere/7 -> Terminator_6/1
  atmosphere/6 -> Terminator_5/1
  atmosphere/5 -> Terminator_4/1
  atmosphere/3 -> Terminator_3/1
  atmosphere/2 -> Terminator_2/1
  atmosphere/1 -> Terminator_1/1
  Mux/1 -> Fgr transformation/1
  "x "/1 -> Mux/1
  Fgr transformation/1 -> Fgr/1
  mass cg inertia/1 -> W/1
  massinit/1 -> mass cg inertia/1
  yatm/1 -> atmosphere/1
  W/1 -> Mux1/3
  Mux1/1 -> Mux/2
  zero/1 -> Mux1/1, Mux1/2
  atmosphere/4 -> W/2

== system Citation_2017a/Cessna Citation 500/Citation model DASMAT/AIRCRAFT MODEL/LANDING GEAR ==
  note: Landing Gear Model
      | Cessna Citation 500
      | Version 0.04NLR
      | (c) A.R. Veldhuijzen September 2001
  x : Inport
  xdot : Inport  Port=2
  massinit : Inport  Port=3
  ua : Inport  Port=4
  terr elev : Inport  Port=5
  Gear axes-cg transformation : Subsystem
  Landing Gear model : Subsystem
  Switch : Switch  Threshold=0.95  SaturateOnIntegerOverflow=on
  gear position : Selector  IndexOptions=Index vector (dialog)  Indices=[8]  OutputSizes=1
  zero : Constant  Value=[0 0 0 0 0 0]
  Fmt : Outport
  wires:
  xdot/1 -> Landing Gear model/2(xdot)
  x/1 -> Landing Gear model/1(x), Gear axes-cg transformation/2("x ")
  massinit/1 -> Gear axes-cg transformation/3(massinit)
  Gear axes-cg transformation/1(FMt) -> Fmt/1
  zero/1 -> Switch/1
  Landing Gear model/1(Forces and Moments) -> Switch/3
  Switch/1 -> Gear axes-cg transformation/1(FMt model)
  ua/1 -> gear position/1
  gear position/1 -> Switch/2
  terr elev/1 -> Landing Gear model/3(terrain elevation)

== system Citation_2017a/Cessna Citation 500/Citation model DASMAT/AIRCRAFT MODEL/OBSERVATIONS ==
  note: Modified by Alex : Flight-Path Subsystem from Ac_mod instead of Ac_modpc
  x : Inport
  xdot : Inport  Port=2
  yuvw : Inport  Port=3
  FMtot : Inport  Port=4
  FMa : Inport  Port=5
  Fgr : Inport  Port=6
  massinit : Inport  Port=7
  yatm : Inport  Port=8
  Acceleration : Subsystem
  Energy : Subsystem
  Flight-Path : Subsystem
  yacc : Outport
  yfp : Outport  Port=2
  ys : Outport  Port=3
  wires:
  yuvw/1 -> Flight-Path/3(yuvw)
  Flight-Path/1(yfp) -> yfp/1
  Energy/1(ys) -> ys/1
  Acceleration/1(yacc) -> yacc/1
  FMa/1 -> Acceleration/4(FMa)
  Fgr/1 -> Acceleration/5(Fgr)
  yatm/1 -> Energy/3(yatm)
  FMtot/1 -> Acceleration/3(FMtot)
  Acceleration/2(acc earth) -> Flight-Path/4(acc earth)
  x/1 -> Flight-Path/1(x), Energy/1(x), Acceleration/1(x)
  xdot/1 -> Flight-Path/2(xdot), Energy/2(xdot), Acceleration/2(xdot)
  massinit/1 -> Acceleration/6(massinit)

== system Citation_2017a/Cessna Citation 500/Citation model DASMAT/AIRCRAFT MODEL/WIND//TURBULENCE ==
  "x " : Inport
  Logarithmic Wind model : Subsystem
  Mux : Mux  Inputs=[12 3]
  Vwind transformation : S-Function  FunctionName=ac_axes  Parameters=3  SFunctionDeploymentMode=off  EnableBusSupport=off
  wind : Outport
  wires:
  Mux/1 -> Vwind transformation/1
  Vwind transformation/1 -> wind/1
  "x "/1 -> Mux/1, Logarithmic Wind model/1(In1)
  Logarithmic Wind model/1(Out1) -> Mux/2

== system Citation_2017a/Pilot/Joystick/DualShock/Add deadzone  ==
  note: Add or subtract deadzone value
  note: Check sign
  "Value " : Inport
  "Input " : Inport  Port=2
  Product : Product
  Sign : Signum
  Sum4 : Sum  Inputs=|++
  Out1 : Outport
  wires:
  "Input "/1 -> Sign/1, Sum4/2
  Product/1 -> Sum4/1
  "Value "/1 -> Product/1
  Sum4/1 -> Out1/1
  Sign/1 -> Product/2

== system Citation_2017a/Pilot/Joystick/DualShock/Add deadzone 1 ==
  note: Check sign
  note: Add or subtract deadzone value
  "Value " : Inport
  "Input " : Inport  Port=2
  Product : Product
  Sign : Signum
  Sum4 : Sum  Inputs=|++
  Out1 : Outport
  wires:
  Sign/1 -> Product/2
  Sum4/1 -> Out1/1
  "Value "/1 -> Product/1
  Product/1 -> Sum4/1
  "Input "/1 -> Sum4/2, Sign/1

== system Citation_2017a/Pilot/Joystick/DualShock/Add deadzone 2 ==
  note: Add or subtract deadzone value
  note: Check sign
  "Value " : Inport
  "Input " : Inport  Port=2
  Product : Product
  Sign : Signum
  Sum4 : Sum  Inputs=|++
  Out1 : Outport
  wires:
  "Input "/1 -> Sign/1, Sum4/2
  Product/1 -> Sum4/1
  "Value "/1 -> Product/1
  Sum4/1 -> Out1/1
  Sign/1 -> Product/2

== system Citation_2017a/Pilot/Joystick/DualShock/Add deadzone 3 ==
  note: Check sign
  note: Add or subtract deadzone value
  "Value " : Inport
  "Input " : Inport  Port=2
  Product : Product
  Sign : Signum
  Sum4 : Sum  Inputs=|++
  Out1 : Outport
  wires:
  Sign/1 -> Product/2
  Sum4/1 -> Out1/1
  "Value "/1 -> Product/1
  Product/1 -> Sum4/1
  "Input "/1 -> Sum4/2, Sign/1

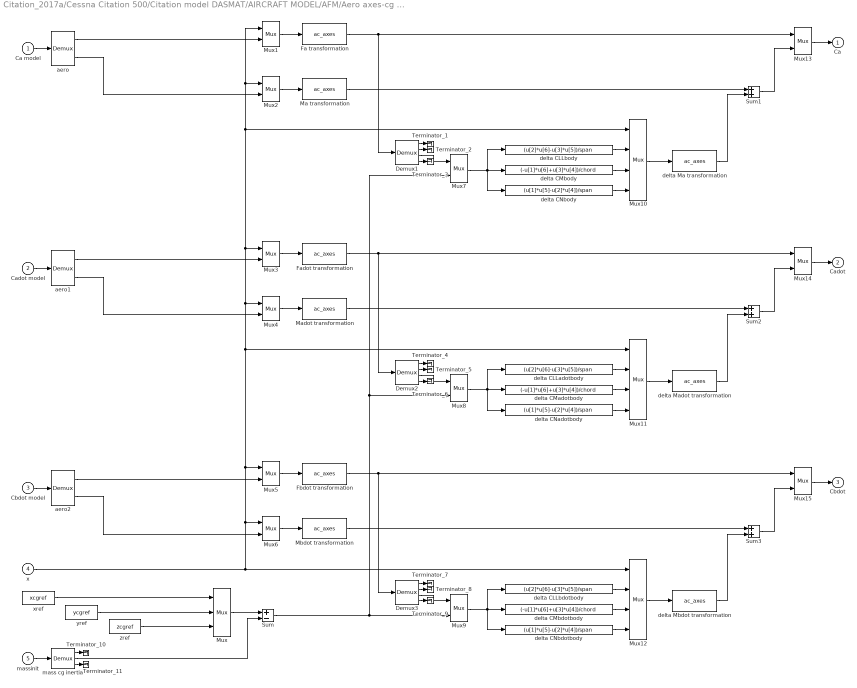
== system Citation_2017a/Cessna Citation 500/Citation model DASMAT/AIRCRAFT MODEL/AFM/Aero axes-cg transformation ==
  Ca model : Inport
  Cadot model : Inport  Port=2
  Cbdot model : Inport  Port=3
  "x " : Inport  Port=4
  massinit : Inport  Port=5
  Demux1 : Demux  Outputs=[3 3 3 3]
  Demux2 : Demux  Outputs=[3 3 3 3]
  Demux3 : Demux  Outputs=[3 3 3 3]
  Fa transformation : S-Function  FunctionName=ac_axes  Parameters=axes_CFMaero  SFunctionDeploymentMode=off  EnableBusSupport=off
  Fadot transformation : S-Function  FunctionName=ac_axes  Parameters=axes_CFMaero  SFunctionDeploymentMode=off  EnableBusSupport=off
  Fbdot transformation : S-Function  FunctionName=ac_axes  Parameters=axes_CFMaero  SFunctionDeploymentMode=off  EnableBusSupport=off
  Ma transformation : S-Function  FunctionName=ac_axes  Parameters=axes_CFMaero  SFunctionDeploymentMode=off  EnableBusSupport=off
  Madot transformation : S-Function  FunctionName=ac_axes  Parameters=axes_CFMaero  SFunctionDeploymentMode=off  EnableBusSupport=off
  Mbdot transformation : S-Function  FunctionName=ac_axes  Parameters=axes_CFMaero  SFunctionDeploymentMode=off  EnableBusSupport=off
  Mux : Mux  Inputs=3
  Mux{1..6} (6 alike) : Mux  Inputs=[12 3]
  Mux10 : Mux  Inputs=[12 1 1 1]
  Mux11 : Mux  Inputs=[12 1 1 1]
  Mux12 : Mux  Inputs=[12 1 1 1]
  Mux13 : Mux  Inputs=[12 12]
  Mux14 : Mux  Inputs=[12 12]
  Mux15 : Mux  Inputs=[12 12]
  Mux7 : Mux  Inputs=[3 3]
  Mux8 : Mux  Inputs=[3 3]
  Mux9 : Mux  Inputs=[3 3]
  Sum : Sum  Inputs=+-  SaturateOnIntegerOverflow=on  InputSameDT=on  OutDataTypeStr=Inherit: Same as first input
  Sum1 : Sum  SaturateOnIntegerOverflow=on  InputSameDT=on  OutDataTypeStr=Inherit: Same as first input
  Sum2 : Sum  SaturateOnIntegerOverflow=on  InputSameDT=on  OutDataTypeStr=Inherit: Same as first input
  Sum3 : Sum  SaturateOnIntegerOverflow=on  InputSameDT=on  OutDataTypeStr=Inherit: Same as first input
  Terminator_{1..11} (11 alike) : Terminator
  aero : Demux  Outputs=[3 3]
  aero1 : Demux  Outputs=[3 3]
  aero2 : Demux  Outputs=[3 3]
  delta CLLadotbody : Fcn  Expr=(u[2]*u[6]-u[3]*u[5])/span
  delta CLLbdotbody : Fcn  Expr=(u[2]*u[6]-u[3]*u[5])/span
  delta CLLbody : Fcn  Expr=(u[2]*u[6]-u[3]*u[5])/span
  delta CMadotbody : Fcn  Expr=(-u[1]*u[6]+u[3]*u[4])/chord
  delta CMbdotbody : Fcn  Expr=(-u[1]*u[6]+u[3]*u[4])/chord
  delta CMbody : Fcn  Expr=(-u[1]*u[6]+u[3]*u[4])/chord
  delta CNadotbody : Fcn  Expr=(u[1]*u[5]-u[2]*u[4])/span
  delta CNbdotbody : Fcn  Expr=(u[1]*u[5]-u[2]*u[4])/span
  delta CNbody : Fcn  Expr=(u[1]*u[5]-u[2]*u[4])/span
  delta Ma transformation : S-Function  FunctionName=ac_axes  Parameters=2  SFunctionDeploymentMode=off  EnableBusSupport=off
  delta Madot transformation : S-Function  FunctionName=ac_axes  Parameters=2  SFunctionDeploymentMode=off  EnableBusSupport=off
  delta Mbdot transformation : S-Function  FunctionName=ac_axes  Parameters=2  SFunctionDeploymentMode=off  EnableBusSupport=off
  mass cg inertia : Demux  Outputs=[1 3 4]
  xref : Constant  Value=xcgref
  yref : Constant  Value=ycgref
  zref : Constant  Value=zcgref
  Ca : Outport
  Cadot : Outport  Port=2
  Cbdot : Outport  Port=3
  wires:
  mass cg inertia/3 -> Terminator_11/1
  mass cg inertia/1 -> Terminator_10/1
  Demux3/4 -> Terminator_9/1
  Demux3/2 -> Terminator_8/1
  Demux3/1 -> Terminator_7/1
  Demux2/4 -> Terminator_6/1
  Demux2/2 -> Terminator_5/1
  Demux2/1 -> Terminator_4/1
  Demux1/4 -> Terminator_3/1
  Demux1/2 -> Terminator_2/1
  Demux1/1 -> Terminator_1/1
  aero1/1 -> Mux3/2
  Cadot model/1 -> aero1/1
  aero1/2 -> Mux4/2
  Ca model/1 -> aero/1
  massinit/1 -> mass cg inertia/1
  aero/1 -> Mux1/2
  xref/1 -> Mux/1
  yref/1 -> Mux/2
  zref/1 -> Mux/3
  mass cg inertia/2 -> Sum/2
  Mux/1 -> Sum/1
  Fa transformation/1 -> Demux1/1, Mux13/1
  Mux7/1 -> delta CLLbody/1, delta CNbody/1, delta CMbody/1
  delta CLLbody/1 -> Mux10/2
  delta CMbody/1 -> Mux10/3
  delta CNbody/1 -> Mux10/4
  Mux10/1 -> delta Ma transformation/1
  Ma transformation/1 -> Sum1/1
  Sum1/1 -> Mux13/2
  Mux13/1 -> Ca/1
  Mux1/1 -> Fa transformation/1
  Mux3/1 -> Fadot transformation/1
  Mux14/1 -> Cadot/1
  Sum2/1 -> Mux14/2
  Madot transformation/1 -> Sum2/1
  Mux12/1 -> delta Mbdot transformation/1
  delta CNbdotbody/1 -> Mux12/4
  delta CMbdotbody/1 -> Mux12/3
  delta CLLbdotbody/1 -> Mux12/2
  Mux9/1 -> delta CLLbdotbody/1, delta CNbdotbody/1, delta CMbdotbody/1
  Mux4/1 -> Madot transformation/1
  Mux2/1 -> Ma transformation/1
  aero/2 -> Mux2/2
  delta Ma transformation/1 -> Sum1/2
  Demux1/3 -> Mux7/1
  Demux3/3 -> Mux9/1
  Demux2/3 -> Mux8/1
  Mux11/1 -> delta Madot transformation/1
  delta CNadotbody/1 -> Mux11/4
  delta CMadotbody/1 -> Mux11/3
  delta CLLadotbody/1 -> Mux11/2
  Mux8/1 -> delta CLLadotbody/1, delta CNadotbody/1, delta CMadotbody/1
  Fadot transformation/1 -> Demux2/1, Mux14/1
  delta Madot transformation/1 -> Sum2/2
  Sum/1 -> Mux8/2, Mux7/2, Mux9/2
  Mux6/1 -> Mbdot transformation/1
  Mux5/1 -> Fbdot transformation/1
  aero2/2 -> Mux6/2
  Cbdot model/1 -> aero2/1
  aero2/1 -> Mux5/2
  "x "/1 -> Mux4/1, Mux3/1, Mux2/1, Mux1/1, Mux10/1, Mux11/1, Mux5/1, Mux6/1, Mux12/1
  Mbdot transformation/1 -> Sum3/1
  Fbdot transformation/1 -> Demux3/1, Mux15/1
  Sum3/1 -> Mux15/2
  delta Mbdot transformation/1 -> Sum3/2
  Mux15/1 -> Cbdot/1

== system Citation_2017a/Cessna Citation 500/Citation model DASMAT/AIRCRAFT MODEL/AFM/Aeromod ==
  x : Inport
  ua : Inport  Port=2
  massinit : Inport  Port=3
  yad1 : Inport  Port=4
  yad2 : Inport  Port=5
  gust : Inport  Port=6
  yatm : Inport  Port=7
  Demux : Demux  Outputs=[6 6 6 6]
  Mux1 : Mux  Inputs=24
  SubSystem : Subsystem
  cg selector : Selector  IndexOptions=Index vector (dialog)  Indices=[2 3 4]  OutputSizes=1
  Ca : Outport
  Cadot : Outport  Port=2
  Cbdot : Outport  Port=3
  Cag : Outport  Port=4
  wires:
  Mux1/1 -> Demux/1
  Demux/1 -> Ca/1
  Demux/2 -> Cadot/1
  Demux/3 -> Cbdot/1
  Demux/4 -> Cag/1
  SubSystem/2(CY) -> Mux1/2
  SubSystem/3(CZ) -> Mux1/3
  SubSystem/5(CM) -> Mux1/5
  SubSystem/6(CN) -> Mux1/6
  SubSystem/8(CYadot) -> Mux1/8
  SubSystem/9(CZadot) -> Mux1/9
  SubSystem/11(CMadot) -> Mux1/11
  SubSystem/12(CNadot) -> Mux1/12
  SubSystem/14(CYbdot) -> Mux1/14
  SubSystem/15(CZbdot) -> Mux1/15
  SubSystem/17(CMbdot) -> Mux1/17
  SubSystem/18(CNbdot) -> Mux1/18
  SubSystem/20(CYg) -> Mux1/20
  SubSystem/21(CZg) -> Mux1/21
  SubSystem/23(CMg) -> Mux1/23
  SubSystem/24(CNg) -> Mux1/24
  SubSystem/22(CLLg) -> Mux1/22
  SubSystem/19(CXg) -> Mux1/19
  SubSystem/16(CLLbdot) -> Mux1/16
  SubSystem/13(CXbdot) -> Mux1/13
  SubSystem/10(CLLadot) -> Mux1/10
  SubSystem/7(CXadot) -> Mux1/7
  SubSystem/4(CLL) -> Mux1/4
  SubSystem/1(CX) -> Mux1/1
  massinit/1 -> cg selector/1
  yad1/1 -> SubSystem/4(yad1)
  gust/1 -> SubSystem/6(gust)
  yad2/1 -> SubSystem/5(yad2)
  ua/1 -> SubSystem/2(ua)
  x/1 -> SubSystem/1(x)
  cg selector/1 -> SubSystem/3(cg)
  yatm/1 -> SubSystem/7(yatm)

== system Citation_2017a/Cessna Citation 500/Citation model DASMAT/AIRCRAFT MODEL/AFM/FMaerodims ==
  Ca : Inport
  Cadot : Inport  Port=2
  Cbdot : Inport  Port=3
  x : Inport  Port=4
  yad1 : Inport  Port=5
  Prod : Product  SaturateOnIntegerOverflow=on  InputSameDT=on  OutDataTypeStr=Inherit: Same as first input
  Prod1 : Product  Inputs=3  SaturateOnIntegerOverflow=on  InputSameDT=on  OutDataTypeStr=Inherit: Same as first input
  Prod2 : Product  Inputs=3  SaturateOnIntegerOverflow=on  InputSameDT=on  OutDataTypeStr=Inherit: Same as first input
  b/V : Fcn  Expr=span/u[4]
  c/V : Fcn  Expr=chord/u[4]
  dims : Subsystem
  dims1 : Subsystem
  dims2 : Subsystem
  qdyn*S : Fcn  Expr=u[2]*S
  FMa : Outport
  FMadot : Outport  Port=2
  FMbdot : Outport  Port=3
  wires:
  Ca/1 -> Prod/1
  Prod/1 -> dims/1(FM/length)
  dims/1(FM) -> FMa/1
  yad1/1 -> qdyn*S/1
  Cbdot/1 -> Prod2/1
  qdyn*S/1 -> Prod2/2, Prod1/2, Prod/2
  Cadot/1 -> Prod1/1
  Prod1/1 -> dims1/1(F FM/length)
  dims1/1(FM) -> FMadot/1
  Prod2/1 -> dims2/1(F FM/length)
  dims2/1(FM) -> FMbdot/1
  x/1 -> b/V/1, c/V/1
  c/V/1 -> Prod1/3
  b/V/1 -> Prod2/3

== system Citation_2017a/Cessna Citation 500/Citation model DASMAT/AIRCRAFT MODEL/AFM/FMgustdims ==
  Cag : Inport
  yad1 : Inport  Port=2
  Prod : Product  SaturateOnIntegerOverflow=on  InputSameDT=on  OutDataTypeStr=Inherit: Same as first input
  dims : Subsystem
  qdyn*S : Fcn  Expr=u[2]*S
  FMag : Outport
  wires:
  Cag/1 -> Prod/1
  Prod/1 -> dims/1(F M/length)
  yad1/1 -> qdyn*S/1
  dims/1(FM) -> FMag/1
  qdyn*S/1 -> Prod/2

== system Citation_2017a/Cessna Citation 500/Citation model DASMAT/AIRCRAFT MODEL/AFM/Gust axes-cg transformation ==
  Cag model : Inport
  "x " : Inport  Port=2
  massinit : Inport  Port=3
  Demux1 : Demux  Outputs=[3 3 3 3]
  Fag transformation : S-Function  FunctionName=ac_axes  Parameters=axes_CFMgust  SFunctionDeploymentMode=off  EnableBusSupport=off
  Mag transformation : S-Function  FunctionName=ac_axes  Parameters=axes_CFMgust  SFunctionDeploymentMode=off  EnableBusSupport=off
  Mux1 : Mux  Inputs=[12 3]
  Mux2 : Mux  Inputs=[12 3]
  Mux3 : Mux  Inputs=[3 3]
  Mux4 : Mux  Inputs=[12 1 1 1]
  Mux5 : Mux  Inputs=[12 12]
  Mux6 : Mux  Inputs=3
  Sum : Sum  Inputs=+-  SaturateOnIntegerOverflow=on  InputSameDT=on  OutDataTypeStr=Inherit: Same as first input
  Sum1 : Sum  SaturateOnIntegerOverflow=on  InputSameDT=on  OutDataTypeStr=Inherit: Same as first input
  Terminator_{1..5} (5 alike) : Terminator
  delta CLLbody : Fcn  Expr=(u[2]*u[6]-u[3]*u[5])/span
  delta CMbody : Fcn  Expr=(-u[1]*u[6]+u[3]*u[4])/chord
  delta CNbody : Fcn  Expr=(u[1]*u[5]-u[2]*u[4])/span
  delta Mag transformation : S-Function  FunctionName=ac_axes  Parameters=2  SFunctionDeploymentMode=off  EnableBusSupport=off
  gust : Demux  Outputs=[3 3]
  mass cg inertia : Demux  Outputs=[1 3 4]
  xref : Constant  Value=xcgref
  yref : Constant  Value=ycgref
  zref : Constant  Value=zcgref
  Cag : Outport
  wires:
  mass cg inertia/3 -> Terminator_5/1
  mass cg inertia/1 -> Terminator_4/1
  Demux1/4 -> Terminator_3/1
  Demux1/2 -> Terminator_2/1
  Demux1/1 -> Terminator_1/1
  Cag model/1 -> gust/1
  massinit/1 -> mass cg inertia/1
  gust/1 -> Mux1/2
  xref/1 -> Mux6/1
  yref/1 -> Mux6/2
  zref/1 -> Mux6/3
  mass cg inertia/2 -> Sum/2
  Mux6/1 -> Sum/1
  Fag transformation/1 -> Demux1/1, Mux5/1
  Mag transformation/1 -> Sum1/1
  Sum1/1 -> Mux5/2
  Mux5/1 -> Cag/1
  Mux1/1 -> Fag transformation/1
  delta Mag transformation/1 -> Sum1/2
  Mux2/1 -> Mag transformation/1
  Sum/1 -> Mux3/2
  gust/2 -> Mux2/2
  "x "/1 -> Mux2/1, Mux1/1, Mux4/1
  Mux3/1 -> delta CLLbody/1, delta CNbody/1, delta CMbody/1
  delta CLLbody/1 -> Mux4/2
  delta CMbody/1 -> Mux4/3
  delta CNbody/1 -> Mux4/4
  Demux1/3 -> Mux3/1
  Mux4/1 -> delta Mag transformation/1
